simulink library "wind2D_cl"  (R2020a)
settings: Solver=VariableStepAuto  StartTime=0.0  StopTime=10.0  RelTol=1e-3
undefined symbols (not defined in the file): Env
libraries: AirDensity_ul x1, LinWindVel2D_ul x1, StopSim_ul x1
settings Model: Creator=jbore  LastModifiedBy=John Jr
settings SFSimCC: CustomCodeUndefinedFunction=UseInterfaceOnly

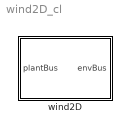
== system wind2D_cl ==
  wind2D : Subsystem

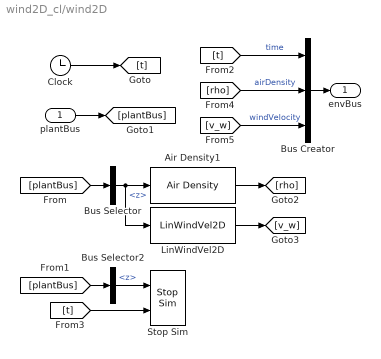
== system wind2D_cl/wind2D ==
  plantBus : Inport
  Air Density1 : AirDensity_ul/Air Density  rho=Env.density.Value  g=Env.grav.Value  M=Env.M.Value  R=Env.R.Value  T_0=Env.temp.Value
  Bus Creator : BusCreator  Inputs=3
  Bus Selector : BusSelector  OutputSignals=z
  Bus Selector2 : BusSelector  OutputSignals=z
  Clock : Clock
  LinWindVel2D : LinWindVel2D_ul/LinWindVel2D  v0=Env.wind0.Value  m=Env.windSlope.Value
  Stop Sim : StopSim_ul/Stop Sim  z_0=Env.gndAlt.Value  t_b=Mot.t_b
  envBus : Outport  VectorParamsAs1DForOutWhenUnconnected=off
  wires:
  Bus Creator/1 -> envBus/1
  Clock/1 -> [t]
  [t] -> Bus Creator/1  "time"
  plantBus/1 -> [plantBus]
  [plantBus] -> Bus Selector/1
  Bus Selector/1 -> LinWindVel2D/1, Air Density1/1  "<z>"
  Air Density1/1 -> [rho]
  [rho] -> Bus Creator/2  "airDensity"
  [plantBus] -> Bus Selector2/1
  Bus Selector2/1 -> Stop Sim/1  "<z>"
  [t] -> Stop Sim/2
  LinWindVel2D/1 -> [v_w]
  [v_w] -> Bus Creator/3  "windVelocity"
